simulink model "ukladRLC"  (Simulink 6.6)
settings: Solver=ode113  StartTime=0.0  StopTime=0.001  RelTol=1e-3
values from neighbouring files (symbols this model uses):
  C = 1e-6    (= 1e-06)    [uklad.m]    (also in uklad2.m; ukladRLC.m)
  L = 1e-3    (= 0.001)    [uklad2.m]    (also in ukladRLC.m)
  R = 1000    [uklad.m]    (also in uklad2.m = 10; ukladRLC.m = 10)
settings Model: Creator=Student  LastModifiedBy=Student

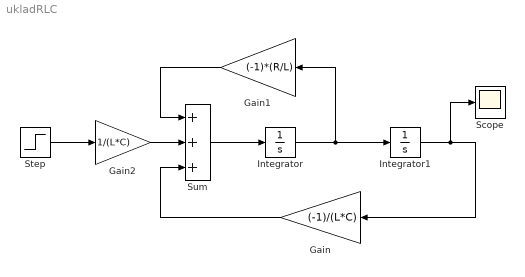
== system ukladRLC ==
  Gain : Gain  Orientation=left  Gain=(-1)/(L*C)
  Gain1 : Gain  Orientation=left  Gain=(-1)*(R/L)
  Gain2 : Gain  Gain=1/(L*C)
  Integrator : Integrator
  Integrator1 : Integrator
  Scope : Scope
      settings: TimeRange=1  YMin=-1  YMax=1
  Step : Step  Time=0.001e-3  SampleTime=0
  Sum : Sum  Inputs=+++
  wires:
  Sum/1 -> Integrator/1
  Integrator/1 -> Integrator1/1, Gain1/1
  Integrator1/1 -> Gain/1, Scope/1
  Gain2/1 -> Sum/2
  Gain1/1 -> Sum/1
  Gain/1 -> Sum/3
  Step/1 -> Gain2/1
